simulink model "TP2"  (R2017b)
settings: Solver=ode23t  StartTime=0.0  StopTime=2.0  RelTol=1e-3
InitFcn:
  | TP2_config
StartFcn:
  | TP2_config
values from neighbouring files (symbols this model uses):
  b = 8.5E-3    (= 0.0085)    [TP2_config.m]
  J = 0.28    [TP2_config.m]
  K = 0.5093    [TP2_config.m]
  Kd = 0.11    [TP2_config.m]
  KdPos = 0.1    [TP2_config.m]
  Ki = 25    [TP2_config.m]
  KiPos = 20    [TP2_config.m]
  Kp = 6    [TP2_config.m]
  KpPos = 250    [TP2_config.m]
  L = 1.6E-3    (= 0.0016)    [TP2_config.m]
  R = 0.02    [TP2_config.m]
libraries: simulink x1
settings Model: Creator=Table2  LastModifiedBy=Table2

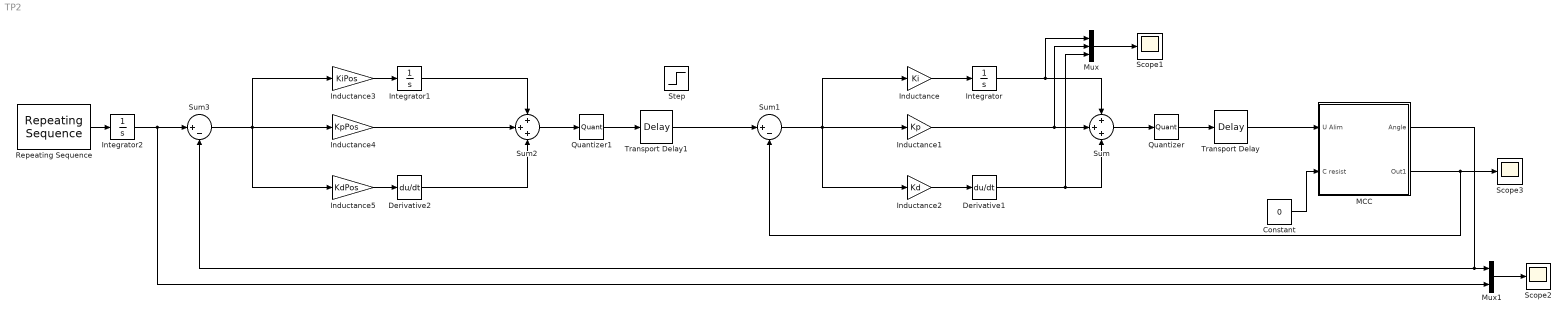
== system TP2 ==
  Constant : Constant  Value=0
  Derivative1 : Derivative  CoefficientInTFapproximation=0.001
  Derivative2 : Derivative  CoefficientInTFapproximation=0.001
  Inductance : Gain  Gain=Ki
  Inductance1 : Gain  Gain=Kp
  Inductance2 : Gain  Gain=Kd
  Inductance3 : Gain  Gain=KiPos
  Inductance4 : Gain  Gain=KpPos
  Inductance5 : Gain  Gain=KdPos
  Integrator : Integrator
  Integrator1 : Integrator
  Integrator2 : Integrator
  MCC : Subsystem
  Mux : Mux  Inputs=3
  Mux1 : Mux  Inputs=3
  Quantizer : Quantizer  QuantizationInterval=0.02
  Quantizer1 : Quantizer  QuantizationInterval=0.02
  Repeating Sequence : simulink/Sources/Repeating Sequence  rep_seq_t=[0 0.1 0.2 0.3 0.8]  rep_seq_y=[0 5 5 0 0]
  Scope1 : Scope
  Scope2 : Scope
  Scope3 : Scope
  Step : Step  Time=0  SampleTime=0
  Sum : Sum  Inputs=+++
  Sum1 : Sum  Inputs=|+-
  Sum2 : Sum  Inputs=+++
  Sum3 : Sum  Inputs=|+-
  Transport Delay : TransportDelay  DelayTime=0.001
  Transport Delay1 : TransportDelay  DelayTime=0.001
  wires:
  Sum/1 -> Quantizer/1
  Inductance1/1 -> Mux/2, Sum/2
  Integrator/1 -> Mux/1, Sum/1
  Inductance/1 -> Integrator/1
  Inductance2/1 -> Derivative1/1
  Derivative1/1 -> Mux/3, Sum/3
  Sum1/1 -> Inductance2/1, Inductance/1, Inductance1/1
  Quantizer/1 -> Transport Delay/1
  Transport Delay/1 -> MCC/1(U Alim)
  Mux/1 -> Scope1/1
  MCC/2(Out1) -> Sum1/2, Scope3/1
  Constant/1 -> MCC/2(C resist)
  Inductance4/1 -> Sum2/2
  Sum2/1 -> Quantizer1/1
  Inductance5/1 -> Derivative2/1
  Inductance3/1 -> Integrator1/1
  Integrator1/1 -> Sum2/1
  Derivative2/1 -> Sum2/3
  Quantizer1/1 -> Transport Delay1/1
  Repeating Sequence/1 -> Integrator2/1
  Sum3/1 -> Inductance5/1, Inductance3/1, Inductance4/1
  MCC/1(Angle) -> Mux1/1, Sum3/2
  Transport Delay1/1 -> Sum1/1
  Mux1/1 -> Scope2/1
  Integrator2/1 -> Mux1/3, Sum3/1

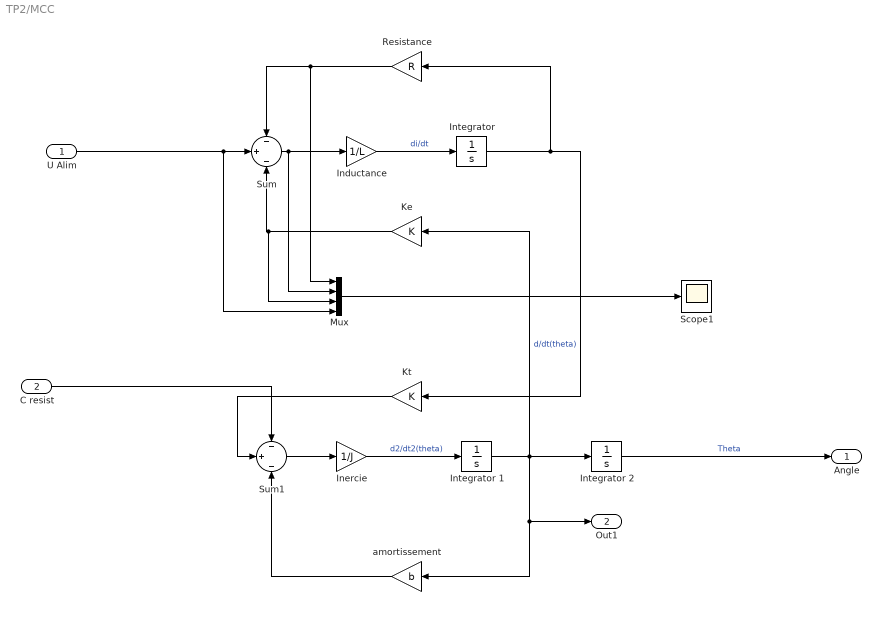
== system TP2/MCC ==
  U Alim : Inport
  C resist : Inport  Port=2
  Inductance : Gain  Gain=1/L
  Inercie : Gain  Gain=1/J
  "Integrator " : Integrator
  Integrator 1 : Integrator
  Integrator 2 : Integrator
  Ke : Gain  Gain=K
  Kt : Gain  Gain=K
  Mux : Mux
  Resistance : Gain  Gain=R
  Scope1 : Scope
  Sum : Sum  Inputs=-|+|-
  Sum1 : Sum  Inputs=-|+|-
  amortissement : Gain  Gain=b
  Angle : Outport
  Out1 : Outport  Port=2
  wires:
  amortissement/1 -> Sum1/3
  Integrator 2/1 -> Angle/1  "Theta"
  Inercie/1 -> Integrator 1/1  "d2/dt2(theta)"
  U Alim/1 -> Mux/4, Sum/2
  Sum/1 -> Mux/2, Inductance/1
  C resist/1 -> Sum1/1
  Sum1/1 -> Inercie/1
  Resistance/1 -> Mux/1, Sum/1
  Mux/1 -> Scope1/1
  "Integrator "/1 -> Resistance/1, Kt/1
  Ke/1 -> Mux/3, Sum/3
  Kt/1 -> Sum1/2
  Integrator 1/1 -> Ke/1, amortissement/1, Out1/1, Integrator 2/1  "d/dt(theta)"
  Inductance/1 -> "Integrator "/1  "di/dt"
